simulink model "untitled1"  (R2023b)
settings: Solver=ode23tb  StartTime=0.0  StopTime=100e-3  MaxStep=Ts  RelTol=1e-3
values from neighbouring files (symbols this model uses):
  alfa = alfap(n)    [FFTalfa.m]    (also in FFTalfa2.m; Parametry.m = 0; WartosciIf.m = 135; WykresyUdcAlfa.m = [0 45 90 135])
  L_obc = 100e-6    (= 0.0001)    [Parametry.m]    (also in WartosciIf.m = 0.2; j60.m; moc.m = 1e-05)
  Lin = Linp(n)    [FFTLin.m]    (also in Parametry.m = 0.003; WykresyUdcLin.m = [100e-6 1e-3 5e-3]; j60.m = 0.005; moc.m = 0.011)
  Ls = 50e-6    (= 5e-05)    [Parametry.m]    (also in moc.m)
  R_obc = 6    [Parametry.m]    (also in moc.m)
  Rin = 1/30*w*Lin    (= 0.0314159265359)    [Parametry.m]    (also in moc.m = 0.115191730632)
undefined symbols (not defined in the file or in its folder): D1, lagging, pulse
libraries: spsSeriesRLCBranchLib x7, spsThyristorLib x6, spsThreePhaseVIMeasurementLib x2, spsCurrentMeasurementLib x1, spsGroundLib x1, spsPLL3phLib x1, spsPulseGeneratorThyristor6PulseLib x1, spsThreePhaseProgrammableVoltageSourceLib x1, spsVoltageMeasurementLib x1, sps_lib x1
settings Model: Creator=rolni  LastModifiedBy=rolni
settings DataIOCC: ReturnWorkspaceOutputs=off

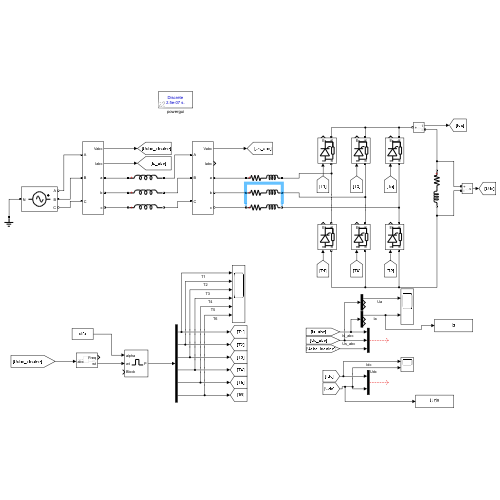
[thumbnail: Simulink's stored preview of the top-level diagram]
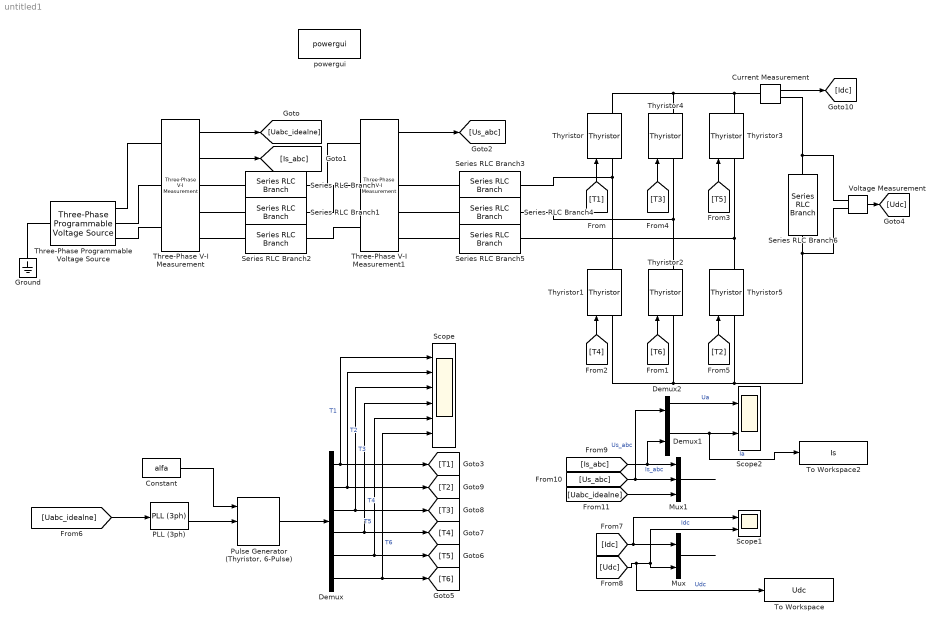
== system untitled1 ==
  Constant : Constant  Value=alfa
  Current Measurement : spsCurrentMeasurementLib/Current Measurement  PhasorSimulation=off  OutputType=Complex  PSBequivalent=0
  Demux : Demux  Outputs=6
  Demux1 : Demux  Outputs=3
  Demux2 : Demux  Outputs=3
  Ground : spsGroundLib/Ground  LConnTagsString=a
  Mux : Mux  Inputs=2
  Mux1 : Mux  Inputs=3
  PLL (3ph) : spsPLL3phLib/PLL (3ph)  Fmin=45  Par_Init=[0, 50]  ParK=[180, 3200, 1]  TcD=1e-4  MaxRateChangeFreq=12  FilterCutOffFreq=25  Ts=0  AGC=on
  "Pulse Generator (Thyristor, 6-Pulse)" : spsPulseGeneratorThyristor6PulseLib/Pulse Generator (Thyristor, 6-Pulse)  GenType=6-pulse  Delta=D1 (lagging)  pwidth=5  Double_Pulse=on  Ts=0
      settings: LibrarySourceBlock=|
      | sps_lib/Power Electronics/Power Electronics Control/Pulse Generator
      | (Thyristor, 6-Pulse)
  Scope : Scope  NumInputPorts=6
  Scope1 : Scope  NumInputPorts=2
  Scope2 : Scope  NumInputPorts=2
  Series RLC Branch : spsSeriesRLCBranchLib/Series RLC Branch  LConnTagsString=__new0  RConnTagsString=__new0  BranchType=L  Resistance=1  Inductance=Ls  SetiL0=off  InitialCurrent=0  Capacitance=1e-6  Setx0=off  InitialVoltage=0  Measurements=None
  Series RLC Branch1 : spsSeriesRLCBranchLib/Series RLC Branch  LConnTagsString=__new0  RConnTagsString=__new0  BranchType=L  Resistance=1  Inductance=Ls  SetiL0=off  InitialCurrent=0  Capacitance=1e-6  Setx0=off  InitialVoltage=0  Measurements=None
  Series RLC Branch2 : spsSeriesRLCBranchLib/Series RLC Branch  LConnTagsString=__new0  RConnTagsString=__new0  BranchType=L  Resistance=1  Inductance=Ls  SetiL0=off  InitialCurrent=0  Capacitance=1e-6  Setx0=off  InitialVoltage=0  Measurements=None
  Series RLC Branch3 : spsSeriesRLCBranchLib/Series RLC Branch  LConnTagsString=__new0  RConnTagsString=__new0  BranchType=RL  Resistance=Rin  Inductance=Lin  SetiL0=off  InitialCurrent=0  Capacitance=1e-6  Setx0=off  InitialVoltage=0  Measurements=None
  Series RLC Branch4 : spsSeriesRLCBranchLib/Series RLC Branch  LConnTagsString=__new0  RConnTagsString=__new0  BranchType=RL  Resistance=Rin  Inductance=Lin  SetiL0=off  InitialCurrent=0  Capacitance=1e-6  Setx0=off  InitialVoltage=0  Measurements=None
  Series RLC Branch5 : spsSeriesRLCBranchLib/Series RLC Branch  LConnTagsString=__new0  RConnTagsString=__new0  BranchType=RL  Resistance=Rin  Inductance=Lin  SetiL0=off  InitialCurrent=0  Capacitance=1e-6  Setx0=off  InitialVoltage=0  Measurements=None
  Series RLC Branch6 : spsSeriesRLCBranchLib/Series RLC Branch  LConnTagsString=__new0  RConnTagsString=__new0  BranchType=RL  Resistance=R_obc  Inductance=L_obc  SetiL0=off  InitialCurrent=0  Capacitance=1e-6  Setx0=off  InitialVoltage=0  Measurements=None
  Three-Phase Programmable Voltage Source : spsThreePhaseProgrammableVoltageSourceLib/Three-Phase Programmable Voltage Source  PositiveSequence="[400  0 50]"  VariationEntity=None  VariationType=Table of time-amplitude pairs  VariationTypeAlt=Step  VariationStep=0.5  VariationRate=10  VariationMagnitude=0.3  VariationFrequency=2  VariationTiming=[1 2]  VariationPhaseA=off  Amplitudes=[1 0.8 1.2 1.0]  TimeValues=[0 0.1 0.15 0.2]  HarmonicGeneration=off  HarmonicA=[3 0.2 -25 0]  HarmonicB=[2 0.15 35 2]  Timing="[0.05  3]"  BusType=swing  Pref=0  Qref=0  Qmin=-inf  Qmax=inf
  Three-Phase V-I Measurement : spsThreePhaseVIMeasurementLib/Three-Phase V-I Measurement  VoltageMeasurement=phase-to-ground  SetLabelV=off  LabelV=Vabc  Vpu=off  VpuLL=off  CurrentMeasurement=yes  SetLabelI=off  LabelI=Iabc  Ipu=off  Pbase=100e6  Vbase=500e3  OutputType=Complex  PhasorSimulation=off  PSBequivalent=0
  Three-Phase V-I Measurement1 : spsThreePhaseVIMeasurementLib/Three-Phase V-I Measurement  VoltageMeasurement=phase-to-ground  SetLabelV=off  LabelV=Vabc  Vpu=off  VpuLL=off  CurrentMeasurement=yes  SetLabelI=off  LabelI=Iabc  Ipu=off  Pbase=100e6  Vbase=500e3  OutputType=Complex  PhasorSimulation=off  PSBequivalent=0
  Thyristor{,1..5} (6 alike) : spsThyristorLib/Thyristor  Ron=Rdiode  Lon=0  Vf=Vdiode  IC=0  Rs=500  Cs=250e-9  Measurements=on
  To Workspace : ToWorkspace  VariableName=Udc  SaveFormat=Structure With Time  SampleTime=-1
  To Workspace2 : ToWorkspace  VariableName=Is  SaveFormat=Structure With Time  SampleTime=-1
  Voltage Measurement : spsVoltageMeasurementLib/Voltage Measurement  PhasorSimulation=off  OutputType=Complex  PSBequivalent=0
  powergui : sps_lib/powergui  Priority=1  SimulationMode=Discrete  SampleTime=2.5e-07  frequency=60  Iterations=50  frequencyindice=50  Pbase=100e6  ErrMax=1e-4  UnitsV=kV  UnitsW=MW  buscounter=0  FunctionMessages=off  echomessages=off  EnableUseOfTLC=off  CurrentSourceSwitches=off  DisableSnubberDevices=off  DisableRonSwitches=off  DisableVfSwitches=off  DisplayEquations=off  AutomaticDiscreteSolvers=off  SolverType=Tustin/Backward Euler (TBE)  Interpol=off  ExternalGateDelay=off  methode=off  Ts=100  x0status=blocks  SPID=on  SwTol=0  HookPort=off  NonlinearTolerance=1e-4  nMaxIteration=100  ContinueOnMaxIteration=off  RestoreLinks=warning  ResistiveCurrentMeasurement=off  Frange=[0:2:500]  Ylog=off  Xlog=on  ShowGrid=off  save=off  variable=ZData  structure=0  ZoomFFT=off  StartTime=0.0  cycles=1  DisplayStyle=1  fundamental=60  FreqAxis=off  MaxFrequency=1000  frequencyindicesteady=1  RmsSteady=1  display=off
  wires:
  [T1] -> Thyristor/1
  [T4] -> Thyristor1/1
  [T6] -> Thyristor2/1
  [T2] -> Thyristor5/1
  "Pulse Generator (Thyristor, 6-Pulse)"/1 -> Demux/1
  Demux/1 -> Scope/1, [T1]  "T1"
  Demux/2 -> Scope/2, [T2]  "T2"
  Demux/3 -> Scope/3, [T3]  "T3"
  Demux/4 -> Scope/4, [T4]  "T4"
  Demux/5 -> Scope/5, [T5]  "T5"
  Demux/6 -> Scope/6, [T6]  "T6"
  Constant/1 -> "Pulse Generator (Thyristor, 6-Pulse)"/1
  PLL (3ph)/2 -> "Pulse Generator (Thyristor, 6-Pulse)"/2
  [Uabc_idealne] -> PLL (3ph)/1
  Three-Phase V-I Measurement/2 -> [Is_abc]
  Three-Phase V-I Measurement/1 -> [Uabc_idealne]
  Three-Phase V-I Measurement1/1 -> [Us_abc]
  [T3] -> Thyristor4/1
  [T5] -> Thyristor3/1
  Voltage Measurement/1 -> [Udc]
  Current Measurement/1 -> [Idc]
  Mux/1 -> ?
  [Idc] -> Scope1/1, Mux/1  "Idc"
  [Udc] -> To Workspace/1, Mux/2, Scope1/2  "Udc"
  Mux1/1 -> ?
  [Is_abc] -> Demux1/1, Mux1/1  "Is_abc"
  [Us_abc] -> Mux1/2, Demux2/1  "Us_abc"
  [Uabc_idealne] -> Mux1/3
  Demux2/1 -> Scope2/1  "Ua"
  Demux1/1 -> To Workspace2/1, Scope2/2  "Ia"
  connections:
  Ground/LConn1 -- Three-Phase Programmable Voltage Source/LConn1
  Three-Phase Programmable Voltage Source/RConn3 -- Three-Phase V-I Measurement/LConn3
  Three-Phase Programmable Voltage Source/RConn2 -- Three-Phase V-I Measurement/LConn2
  Three-Phase Programmable Voltage Source/RConn1 -- Three-Phase V-I Measurement/LConn1
  Three-Phase V-I Measurement/RConn3 -- Series RLC Branch2/LConn1
  Three-Phase V-I Measurement/RConn2 -- Series RLC Branch1/LConn1
  Three-Phase V-I Measurement/RConn1 -- Series RLC Branch/LConn1
  Series RLC Branch2/RConn1 -- Three-Phase V-I Measurement1/LConn3
  Series RLC Branch1/RConn1 -- Three-Phase V-I Measurement1/LConn2
  Series RLC Branch/RConn1 -- Three-Phase V-I Measurement1/LConn1
  Three-Phase V-I Measurement1/RConn3 -- Series RLC Branch5/LConn1
  Three-Phase V-I Measurement1/RConn2 -- Series RLC Branch4/LConn1
  Three-Phase V-I Measurement1/RConn1 -- Series RLC Branch3/LConn1
  Thyristor1/RConn1 -- Series RLC Branch3/RConn1 -- Thyristor/LConn1
  Thyristor2/RConn1 -- Series RLC Branch4/RConn1 -- Thyristor4/LConn1
  Thyristor5/RConn1 -- Series RLC Branch5/RConn1 -- Thyristor3/LConn1
  Thyristor/RConn1 -- Thyristor3/RConn1 -- Current Measurement/LConn1 -- Thyristor4/RConn1
  Current Measurement/RConn1 -- Voltage Measurement/LConn1 -- Series RLC Branch6/LConn1
  Thyristor1/LConn1 -- Thyristor2/LConn1 -- Thyristor5/LConn1 -- Voltage Measurement/LConn2 -- Series RLC Branch6/RConn1
